simulink model "FM"  (R2017a)
settings: Solver=ode4  StartTime=0.0  StopTime=0.4  FixedStep=0.0001  RelTol=1e-3
libraries: simulink_extras x2
settings Model: Creator=carma  LastModifiedBy=carma

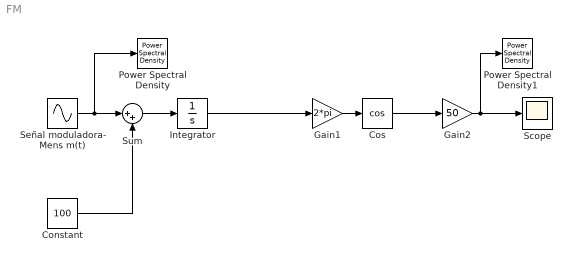
== system FM ==
  Constant : Constant  Value=100
  Cos : Trigonometry  Operator=cos
  Gain1 : Gain  Gain=2*pi
  Gain2 : Gain  Gain=50
  Integrator : Integrator
  Power Spectral Density : simulink_extras/Additional Sinks/Power Spectral Density  npts=512  fftpts=1024  HowOften=64  sampleT=0.001
      settings: SourceProductName=Simulink  SourceProductBaseCode=SL
  Power Spectral Density1 : simulink_extras/Additional Sinks/Power Spectral Density  npts=512  fftpts=1024  HowOften=64  sampleT=0.001
      settings: SourceProductName=Simulink  SourceProductBaseCode=SL
  Scope : Scope
  Señal moduladora- Mens m(t) : Sin  Amplitude=50  Frequency=2*pi*10  SampleTime=0
  Sum : Sum  Inputs=|++
  wires:
  Señal moduladora- Mens m(t)/1 -> Sum/1, Power Spectral Density/1
  Integrator/1 -> Gain1/1
  Gain1/1 -> Cos/1
  Cos/1 -> Gain2/1
  Sum/1 -> Integrator/1
  Constant/1 -> Sum/2
  Gain2/1 -> Power Spectral Density1/1, Scope/1
